simulink model "Simulateur_VRemise_eq06"  (R2024a)
settings: Solver=ode4  StartTime=0.0  StopTime=3  FixedStep=1e-06  RelTol=1e-3
InitFcn:
  | Init
values from neighbouring files (symbols this model uses):
  adL0 = -9.95e-3    (= -0.00995)    [Init.m]    (also in Init_Complet.m = -9.95e-06)
  adL1 = -9.10e-3    (= -0.0091)    [Init.m]    (also in Init_Complet.m = -9.1e-06)
  aKb0 = -1.41e-2    (= -0.0141)    [Init.m]    (also in Init_Complet.m)
  aKb1 = 5.96e-5    (= 5.96e-05)    [Init.m]    (also in Init_Complet.m)
  aL0 = 1.1256e-3    (= 0.0011256)    [Init.m]    (also in Init_Complet.m)
  aL1 = -9.95e-6    (= -9.95e-06)    [Init.m]    (also in Init_Complet.m)
  aL2 = -4.55e-6    (= -4.55e-06)    [Init.m]    (also in Init_Complet.m)
  aPhi0 = -1.41e-2    (= -0.0141)    [Init.m]    (also in Init_Complet.m)
  aPhi1 = 5.96e-5    (= 5.96e-05)    [Init.m]    (also in Init_Complet.m)
  b = 72.82e-3    (= 0.07282)    [Init.m]    (also in Init_Complet.m)
  Ccmax = 5    [Init.m]    (also in Init_Complet.m)
  Ccmin = 0    [Init.m]    (also in Init_Complet.m)
  Ccoff = 2.5    [Init.m]    (also in Init_Complet.m)
  d = 1850    [Init.m]    (also in Init_Complet.m)
  dt = 5e-6    (= 5e-06)    [Init.m]    (also in Init_Complet.m)
  E = 18.6e9    (= 18600000000)    [Init.m]    (also in Init_Complet.m)
  h = 1.46e-3    (= 0.00146)    [Init.m]    (also in Init_Complet.m)
  Imoff = 2.5    [Init.m]    (also in Init_Complet.m)
  K_pwm = 1/5    (= 0.2)    [Init.m]    (also in Init_Complet.m)
  KampL = 1    [Init.m]    (also in Init_Complet.m)
  Kd_pos = 0.00000405    (= 4.05e-06)    [Init.m]    (also in Init_Complet.m = 0.017)
  Ki_i = 180    [Init.m]    (also in Init_Complet.m)
  Ki_pos = 1.2    [Init.m]    (also in Init_Complet.m = 2.8333)
  Km = 1/1.1    (= 0.909090909091)    [Init.m]    (also in Init_Complet.m)
  Kp_i = 0.18    [Init.m]    (also in Init_Complet.m)
  Kp_pos = 0.005    [Init.m]    (also in Init_Complet.m = 0.85)
  Kpos = 205    [Init.m]    (also in Init_Complet.m)
  Kpwmo = 5    [Init.m]    (also in Init_Complet.m)
  Ksh = 1    [Init.m]    (also in Init_Complet.m)
  L = 25e-2    (= 0.25)    [Init.m]    (also in Init_Complet.m)
  M_l_p_b = 0.137    [Init.m]    (also in Init_Complet.m)
  N = 22    [Init.m]    (also in Init_Complet.m)
  Offp = 2.3025    [Init.m]    (also in Init_Complet.m)
  q = 0.14    [Init.m]    (also in Init_Complet.m)
  Rb = 1.63    [Init.m]    (also in Init_Complet.m)
  Ts_p = Ts_reg    (= 1e-06)    [Init.m]    (also in Init_Complet.m = 0.002)
  Vamp_max = 5    [Init.m]    (also in Init_Complet.m)
  Vamp_min = 0    [Init.m]    (also in Init_Complet.m)
  Vmoff = 2.5    [Init.m]    (also in Init_Complet.m)
  Vref = 1.8    [Init.m]    (also in Init_Complet.m)
  zeta = 0.0917    [Init.m]    (also in Init_Complet.m)
libraries: simulink x3, slpidlib x2
settings Model: SimulationMode=accelerator  Creator=jeann  LastModifiedBy=jotur116
settings RTWCC: GPUComputeCapability=3.5

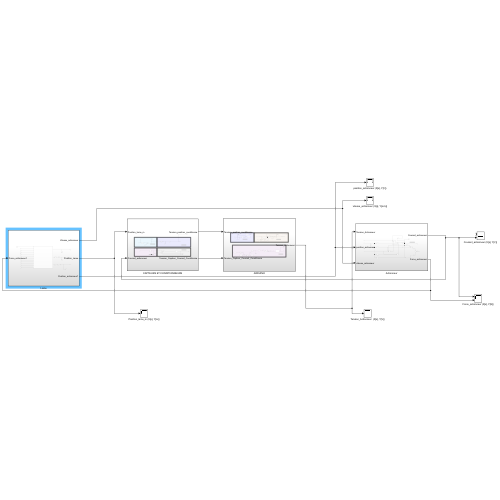
[thumbnail: Simulink's stored preview of the top-level diagram]
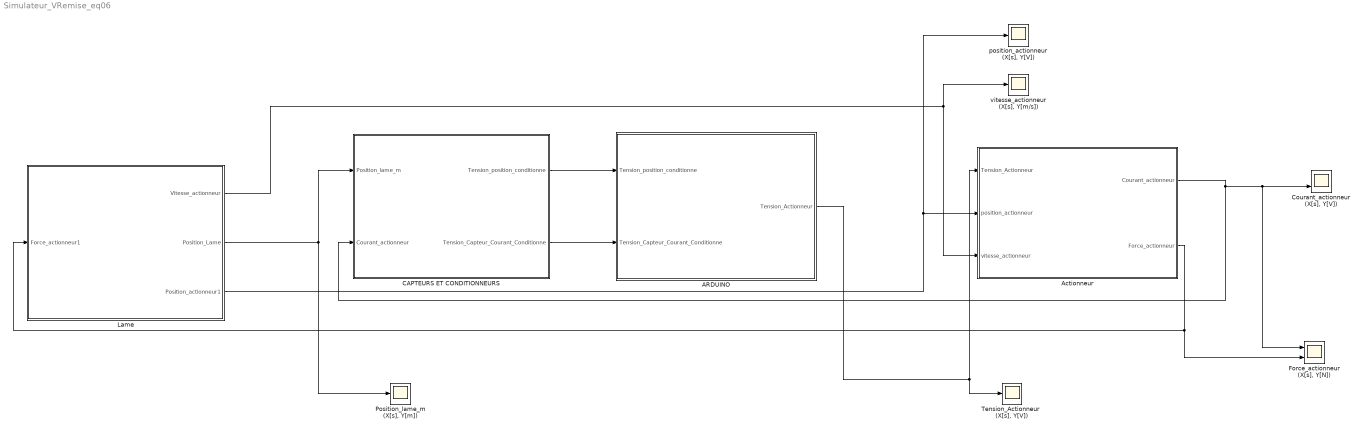
== system Simulateur_VRemise_eq06 ==
  ARDUINO : Subsystem
  Actionneur : Subsystem
  CAPTEURS ET CONDITIONNEURS : Subsystem
  "Courant_actionneur (X[s], Y[V])" : Scope  NumInputPorts=2
  "Force_actionneur (X[s], Y[N])" : Scope  NumInputPorts=2
  Lame : Subsystem
  "Position_lame_m (X[s], Y[m])" : Scope
  "Tension_Actionneur  (X[s], Y[V])" : Scope
  "position_actionneur (X[s], Y[V])" : Scope
  "vitesse_actionneur (X[s], Y[m/s])" : Scope
  wires:
  Lame/3(Position_actionneur1) -> "position_actionneur (X[s], Y[V])"/1, Actionneur/2(position_actionneur)
  Lame/1(Vitesse_actionneur) -> Actionneur/3(vitesse_actionneur), "vitesse_actionneur (X[s], Y[m/s])"/1
  Lame/2(Position_Lame) -> CAPTEURS ET CONDITIONNEURS/1(Position_lame_m), "Position_lame_m (X[s], Y[m])"/1
  CAPTEURS ET CONDITIONNEURS/1(Tension_position_conditionne) -> ARDUINO/1(Tension_position_conditionne)
  CAPTEURS ET CONDITIONNEURS/2(Tension_Capteur_Courant_Conditionne) -> ARDUINO/2(Tension_Capteur_Courant_Conditionne)
  ARDUINO/1(Tension_Actionneur) -> "Tension_Actionneur  (X[s], Y[V])"/1, Actionneur/1(Tension_Actionneur)
  Actionneur/1(Courant_actionneur) -> CAPTEURS ET CONDITIONNEURS/2(Courant_actionneur), "Courant_actionneur (X[s], Y[V])"/2, "Force_actionneur (X[s], Y[N])"/1
  Actionneur/2(Force_actionneur) -> Lame/1(Force_actionneur1), "Force_actionneur (X[s], Y[N])"/2

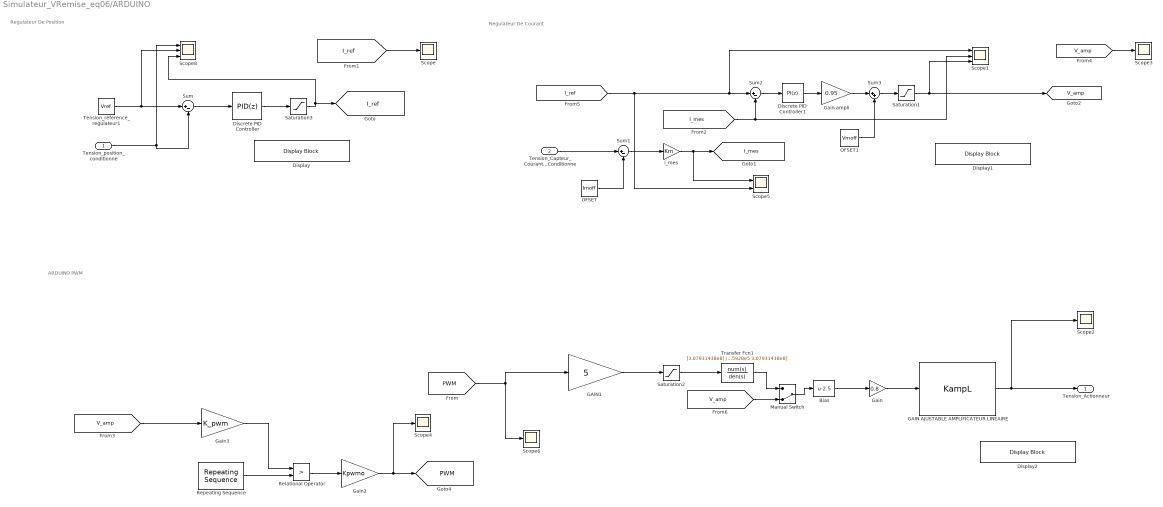
== system Simulateur_VRemise_eq06/ARDUINO ==
  note: Regulateur De Position
  note: Regulateur De Courant
  note: ARDUINO PWM
  Tension_position_conditionne : Inport
  Tension_Capteur_Courant_Conditionne : Inport  Port=2
  Bias : Bias  Bias=-2.5  SaturateOnIntegerOverflow=off
  Discrete PID Controller : slpidlib/PID Controller  Controller=PID  Form=Parallel  TimeDomain=Discrete-time  UseExternalTs=off  SampleTime=Ts_p  IntegratorMethod=Forward Euler  FilterMethod=Forward Euler  ControllerParametersSource=internal  P=Kp_pos  I=Ki_pos  UseKiTs=off  D=Kd_pos  UseExternalDerivativeSource=off  N=100  UseFilter=on  TunerSelectOption=Transfer Function Based (PID Tuner App)  InitialConditionSource=internal  InitialConditionForIntegrator=0  InitialConditionForFilter=0  DifferentiatorICPrevScaledInput=0  ExternalReset=none  TrackingMode=off  Kt=1  LimitOutput=on  SatLimitsSource=internal  UpperSaturationLimit=2.35  LowerSaturationLimit=-2.35  LinearizeAsGain=off  AntiWindupMode=back-calculation  Kb=1  LimitIntegrator=off  UpperIntegratorSaturationLimit=inf  LowerIntegratorSaturationLimit=-inf  POutMin=[]  POutMax=[]  IOutMin=[]  IOutMax=[]  DOutMin=[]  DOutMax=[]  NOutMin=[]  NOutMax=[]  SumOutMin=[]  SumOutMax=[]  SaturationOutMin=[]  SaturationOutMax=[]  PParamMin=[]  PParamMax=[]  IParamMin=[]  IParamMax=[]  DParamMin=[]  DParamMax=[]  NParamMin=[]  NParamMax=[]  KbParamMin=[]  KbParamMax=[]  KtParamMin=[]  KtParamMax=[]  KbOutMin=[]  KbOutMax=[]  KtOutMin=[]  KtOutMax=[]  IntegratorOutMin=[]  IntegratorOutMax=[]  FilterOutMin=[]  FilterOutMax=[]  SumI1OutMin=[]  SumI1OutMax=[]  SumI2OutMin=[]  SumI2OutMax=[]  SumI3OutMin=[]  SumI3OutMax=[]  SumI4OutMin=[]  SumI4OutMax=[]  SumDOutMin=[]  SumDOutMax=[]  DifferentiatorOutMin=[]  DifferentiatorOutMax=[]  FilterDiffOutCoefMin=[]  FilterDiffOutCoefMax=[]  ReciprocalOutMin=[]  ReciprocalOutMax=[]  SumDenOutMin=[]  SumDenOutMax=[]  SumNumOutMin=[]  SumNumOutMax=[]  DivideOutMin=[]  DivideOutMax=[]  UdiffTsProdOutMin=[]  UdiffTsProdOutMax=[]  NTsProdOutMin=[]  NTsProdOutMax=[]  UintegralTsProdOutMin=[]  UintegralTsProdOutMax=[]  UngainTsProdOutMin=[]  UngainTsProdOutMax=[]  ClampingZeroOutDataTypeStr=Inherit: Inherit via back propagation  ClampingZeroOutMin=[]  ClampingZeroOutMax=[]  FilterDenConstantOutDataTypeStr=Inherit: Inherit via back propagation  FilterDenConstantOutMin=[]  FilterDenConstantOutMax=[]  PCopyOutDataTypeStr=Inherit: Inherit via back propagation  PCopyOutMin=[]  PCopyOutMax=[]  NCopyOutDataTypeStr=Inherit: Inherit via back propagation  NCopyOutMin=[]  NCopyOutMax=[]  IntegratorContinuousStateAttributes=''  IntegratorStateMustResolveToSignalObject=off  IntegratorRTWStateStorageClass=Auto  FilterContinuousStateAttributes=''  FilterStateMustResolveToSignalObject=off  FilterRTWStateStorageClass=Auto  ParallelPVariant=InternalParameters  IdealPVariant=Disabled  IVariant=InternalParameters  DVariant=InternalParameters  IntegratorVariant=Discrete  SatVariant=Enabled  AWVariant=BackCalculation  PCopyVariant=Disabled  TRVariant=Disabled  FdbkBlocksVariant=Forward  IdealPFdbkVariant=Disabled  SatFdbkVariant=Disabled  DerivativeFilterVariant=ForwardEulerFilter  NVariant=InternalParameters  NCopyVariant=Disabled  FilterICVariant=InternalICsFilter  IntegratorICVariant=InternalICs  ExternalResetVariant=Disabled  TRSumVariant=Passthrough  SumFdbkVariant=Disabled  SumVariant=Sum_PID  TsampFilterVariant=InternalTs  TsampNgainVariant=Passthrough  TsampIntegralVariant=Disabled_SignalSpec  ExternalSaturationOutDataTypeStr=Inherit: Same as second input  DerivativeSourceVariant=ErrorSignal
      settings: LibrarySourceBlock=simulink/Discrete/Discrete PID Controller
  Discrete PID Controller1 : slpidlib/PID Controller  Controller=PI  Form=Parallel  TimeDomain=Discrete-time  UseExternalTs=off  SampleTime=0.002  IntegratorMethod=Forward Euler  FilterMethod=Forward Euler  ControllerParametersSource=internal  P=Kp_i  I=Ki_i  UseKiTs=off  D=0  UseExternalDerivativeSource=off  N=100  UseFilter=on  TunerSelectOption=Transfer Function Based (PID Tuner App)  InitialConditionSource=internal  InitialConditionForIntegrator=0  InitialConditionForFilter=0  DifferentiatorICPrevScaledInput=0  ExternalReset=none  TrackingMode=off  Kt=1  LimitOutput=off  SatLimitsSource=internal  UpperSaturationLimit=5  LowerSaturationLimit=0  LinearizeAsGain=off  AntiWindupMode=back-calculation  Kb=1  LimitIntegrator=off  UpperIntegratorSaturationLimit=inf  LowerIntegratorSaturationLimit=-inf  POutMin=[]  POutMax=[]  IOutMin=[]  IOutMax=[]  DOutMin=[]  DOutMax=[]  NOutMin=[]  NOutMax=[]  SumOutMin=[]  SumOutMax=[]  SaturationOutMin=[]  SaturationOutMax=[]  PParamMin=[]  PParamMax=[]  IParamMin=[]  IParamMax=[]  DParamMin=[]  DParamMax=[]  NParamMin=[]  NParamMax=[]  KbParamMin=[]  KbParamMax=[]  KtParamMin=[]  KtParamMax=[]  KbOutMin=[]  KbOutMax=[]  KtOutMin=[]  KtOutMax=[]  IntegratorOutMin=[]  IntegratorOutMax=[]  FilterOutMin=[]  FilterOutMax=[]  SumI1OutMin=[]  SumI1OutMax=[]  SumI2OutMin=[]  SumI2OutMax=[]  SumI3OutMin=[]  SumI3OutMax=[]  SumI4OutMin=[]  SumI4OutMax=[]  SumDOutMin=[]  SumDOutMax=[]  DifferentiatorOutMin=[]  DifferentiatorOutMax=[]  FilterDiffOutCoefMin=[]  FilterDiffOutCoefMax=[]  ReciprocalOutMin=[]  ReciprocalOutMax=[]  SumDenOutMin=[]  SumDenOutMax=[]  SumNumOutMin=[]  SumNumOutMax=[]  DivideOutMin=[]  DivideOutMax=[]  UdiffTsProdOutMin=[]  UdiffTsProdOutMax=[]  NTsProdOutMin=[]  NTsProdOutMax=[]  UintegralTsProdOutMin=[]  UintegralTsProdOutMax=[]  UngainTsProdOutMin=[]  UngainTsProdOutMax=[]  ClampingZeroOutDataTypeStr=Inherit: Inherit via back propagation  ClampingZeroOutMin=[]  ClampingZeroOutMax=[]  FilterDenConstantOutDataTypeStr=Inherit: Inherit via back propagation  FilterDenConstantOutMin=[]  FilterDenConstantOutMax=[]  PCopyOutDataTypeStr=Inherit: Inherit via back propagation  PCopyOutMin=[]  PCopyOutMax=[]  NCopyOutDataTypeStr=Inherit: Inherit via back propagation  NCopyOutMin=[]  NCopyOutMax=[]  IntegratorContinuousStateAttributes=''  IntegratorStateMustResolveToSignalObject=off  IntegratorRTWStateStorageClass=Auto  FilterContinuousStateAttributes=''  FilterStateMustResolveToSignalObject=off  FilterRTWStateStorageClass=Auto  ParallelPVariant=InternalParameters  IdealPVariant=Disabled  IVariant=InternalParameters  DVariant=Disabled  IntegratorVariant=Discrete  SatVariant=Disabled  AWVariant=Passthrough  PCopyVariant=Disabled  TRVariant=Disabled  FdbkBlocksVariant=Forward  IdealPFdbkVariant=Disabled  SatFdbkVariant=Disabled  DerivativeFilterVariant=Disabled  NVariant=Disabled  NCopyVariant=Disabled_SignalSpec  FilterICVariant=Disabled  IntegratorICVariant=InternalICs  ExternalResetVariant=Disabled  TRSumVariant=Passthrough  SumFdbkVariant=Disabled  SumVariant=Sum_PI  TsampFilterVariant=InternalTs  TsampNgainVariant=Passthrough  TsampIntegralVariant=Disabled_SignalSpec  ExternalSaturationOutDataTypeStr=Inherit: Same as second input  DerivativeSourceVariant=Disabled
      settings: LibrarySourceBlock=simulink/Discrete/Discrete PID Controller
  Display : DisplayBlock  LabelPosition=Hide  Transparency=1
  Display1 : DisplayBlock  LabelPosition=Hide  Transparency=1
  Display2 : DisplayBlock  LabelPosition=Hide  Transparency=1
  GAIN AJUSTABLE AMPLIFICATEUR LINEAIRE : simulink/Math Operations/Slider Gain  gain=KampL  low=1  high=5
  GAIN1 : Gain  Gain=5
  Gain : Gain  Gain=0.8
  "Gain ampli " : Gain  Gain=0.95
  Gain2 : Gain  Gain=Kpwmo  ParamDataTypeStr=double
  Gain3 : Gain  Gain=K_pwm
  Manual Switch : ManualSwitch  CurrentSetting=0
  OFSET : Constant  Value=Imoff
  OFSET1 : Constant  Value=Vmoff
  Relational Operator : RelationalOperator  Operator=>  OutDataTypeStr=boolean  RndMeth=Simplest  InputSameDT=off
  Repeating Sequence : simulink/Sources/Repeating Sequence  rep_seq_t=[0 3.2e-5 6.4e-5]  rep_seq_y=[0 1 0]
  Saturation1 : Saturate  UpperLimit=Vamp_max  LowerLimit=Vamp_min
  Saturation2 : Saturate  UpperLimit=Vamp_max  LowerLimit=Vamp_min
  Saturation3 : Saturate  UpperLimit=2.35  LowerLimit=-2.35
  Scope{,2..4,6} (5 alike) : Scope
  Scope1 : Scope  NumInputPorts=3
  Scope5 : Scope  NumInputPorts=2
  Scope8 : Scope  NumInputPorts=3
  Sum : Sum  Inputs=|+-
  Sum1 : Sum  Inputs=|+-
  Sum2 : Sum  Inputs=|+-
  Sum3 : Sum  Inputs=|++
  Tension_reference_regulateur1 : Constant  Value=Vref
  Transfer Fcn1 : TransferFcn  Numerator=[3.07931438e8]  Denominator=[1 1.0115928e5 3.07931438e8]
  i_mes : Gain  Gain=Km
  Tension_Actionneur : Outport
  tag scope: I_mes=global, I_ref=global, PWM=global, V_amp=global
  wires:
  [I_ref] -> Scope/1
  Discrete PID Controller/1 -> Saturation3/1
  Sum1/1 -> i_mes/1
  Discrete PID Controller1/1 -> "Gain ampli "/1
  "Gain ampli "/1 -> Sum3/1
  Sum2/1 -> Discrete PID Controller1/1
  i_mes/1 -> Scope5/1, [I_mes]
  [V_amp] -> Scope3/1
  OFSET/1 -> Sum1/2
  OFSET1/1 -> Sum3/2
  Sum3/1 -> Saturation1/1
  Tension_Capteur_Courant_Conditionne/1 -> Sum1/1
  Gain2/1 -> Scope4/1, [PWM]
  Gain3/1 -> Relational Operator/1
  Repeating Sequence/1 -> Relational Operator/2
  Relational Operator/1 -> Gain2/1
  [V_amp] -> Gain3/1
  [PWM] -> Scope6/1, GAIN1/1
  [I_ref] -> Scope5/2, Scope1/1, Sum2/1
  [I_mes] -> Scope1/2, Sum2/2
  Saturation1/1 -> [V_amp], Scope1/3
  Saturation3/1 -> [I_ref], Scope8/3
  GAIN AJUSTABLE AMPLIFICATEUR LINEAIRE/1 -> Tension_Actionneur/1, Scope2/1
  Sum/1 -> Discrete PID Controller/1
  Tension_position_conditionne/1 -> Scope8/1, Sum/2
  Tension_reference_regulateur1/1 -> Scope8/2, Sum/1
  GAIN1/1 -> Saturation2/1
  Saturation2/1 -> Transfer Fcn1/1
  Bias/1 -> Gain/1
  Gain/1 -> GAIN AJUSTABLE AMPLIFICATEUR LINEAIRE/1
  Transfer Fcn1/1 -> Manual Switch/1
  Manual Switch/1 -> Bias/1
  [V_amp] -> Manual Switch/2

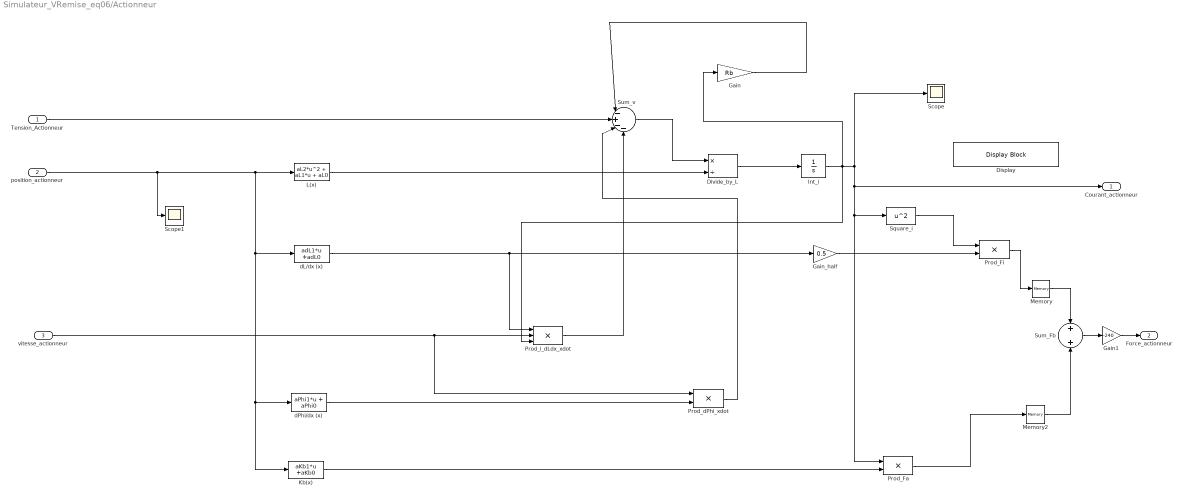
== system Simulateur_VRemise_eq06/Actionneur ==
  Tension_Actionneur : Inport
  position_actionneur : Inport  Port=2
  vitesse_actionneur : Inport  Port=3
  Display : DisplayBlock  LabelPosition=Hide  Transparency=1
  Divide_by_L : Product  Inputs=*/
  Gain : Gain  Gain=Rb
  Gain1 : Gain  Gain=-240
  Gain_half : Gain  Gain=0.5
  Int_i : Integrator
  Kb(x) : Fcn  Expr=aKb1*u +aKb0
  L(x) : Fcn  Expr=aL2*u^2 + aL1*u + aL0
  Memory : Memory
  Memory2 : Memory
  Prod_Fa : Product
  Prod_Fi : Product
  Prod_dPhi_xdot : Product
  Prod_i_dLdx_xdot : Product  Inputs=3
  Scope : Scope
  Scope1 : Scope
  Square_i : Math  Operator=square
  Sum_Fb : Sum
  Sum_v : Sum  Inputs=|-+--
  dL/dx (x) : Fcn  Expr=adL1*u +adL0
  dPhi/dx (x) : Fcn  Expr=aPhi1*u + aPhi0
  Courant_actionneur : Outport
  Force_actionneur : Outport  Port=2
  wires:
  dL/dx (x)/1 -> Gain_half/1, Prod_i_dLdx_xdot/1
  Sum_Fb/1 -> Gain1/1
  Gain/1 -> Sum_v/1
  Prod_i_dLdx_xdot/1 -> Sum_v/4
  L(x)/1 -> Divide_by_L/2
  Square_i/1 -> Prod_Fi/1
  Prod_dPhi_xdot/1 -> Sum_v/3
  Gain_half/1 -> Prod_Fi/2
  dPhi/dx (x)/1 -> Prod_dPhi_xdot/2
  Divide_by_L/1 -> Int_i/1
  Int_i/1 -> Prod_i_dLdx_xdot/3, Courant_actionneur/1, Square_i/1, Prod_Fa/1, Scope/1, Gain/1
  Sum_v/1 -> Divide_by_L/1
  vitesse_actionneur/1 -> Prod_dPhi_xdot/1, Prod_i_dLdx_xdot/2
  Kb(x)/1 -> Prod_Fa/2
  position_actionneur/1 -> Scope1/1, dL/dx (x)/1, Kb(x)/1, dPhi/dx (x)/1, L(x)/1
  Tension_Actionneur/1 -> Sum_v/2
  Prod_Fi/1 -> Memory/1
  Memory/1 -> Sum_Fb/1
  Prod_Fa/1 -> Memory2/1
  Memory2/1 -> Sum_Fb/2
  Gain1/1 -> Force_actionneur/1

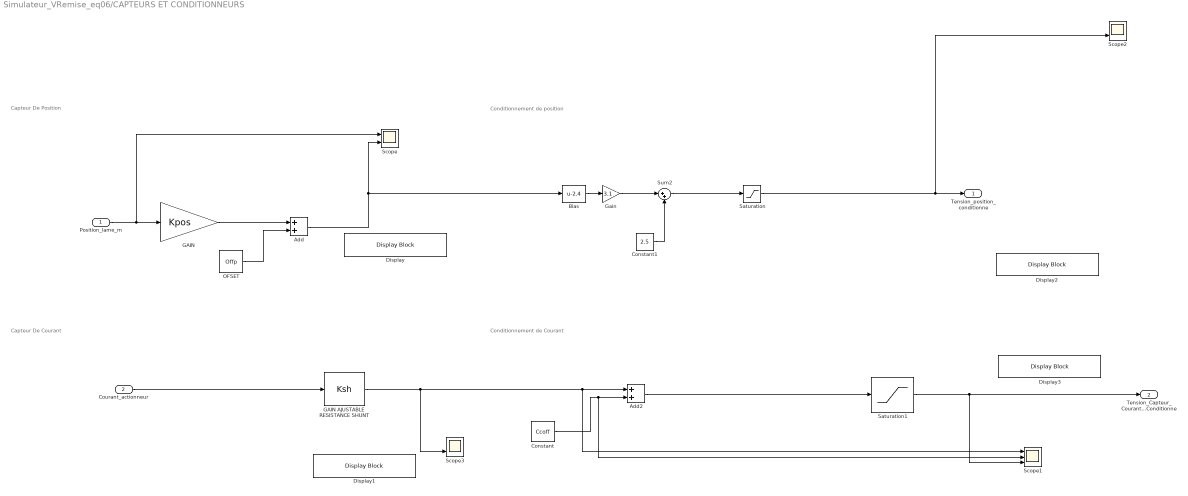
== system Simulateur_VRemise_eq06/CAPTEURS ET CONDITIONNEURS ==
  note: Capteur De Position
  note: Conditionnement de position
  note: Capteur De Courant
  note: Conditionnement de Courant
  Position_lame_m : Inport
  Courant_actionneur : Inport  Port=2
  Add : Sum
  Add2 : Sum
  Bias : Bias  Bias=-2.4  SaturateOnIntegerOverflow=off
  Constant : Constant  Value=Ccoff
  Constant1 : Constant  Value=2.5
  Display{,1..3} (4 alike) : DisplayBlock  LabelPosition=Hide  Transparency=1
  GAIN : Gain  Gain=Kpos
  GAIN AJUSTABLE RESISTANCE SHUNT : simulink/Math Operations/Slider Gain  gain=Ksh  low=1  high=10
  Gain : Gain  Gain=3.1
  OFSET : Constant  Value=Offp
  Saturation : Saturate  UpperLimit=5  LowerLimit=0
  Saturation1 : Saturate  UpperLimit=Ccmax  LowerLimit=Ccmin
  Scope : Scope  NumInputPorts=2
  Scope1 : Scope  NumInputPorts=3
  Scope2 : Scope  NumInputPorts=2
  Scope3 : Scope  NumInputPorts=2
  Sum2 : Sum  Inputs=|++
  Tension_position_conditionne : Outport
  Tension_Capteur_Courant_Conditionne : Outport  Port=2
  wires:
  GAIN/1 -> Add/1
  OFSET/1 -> Add/2
  Saturation1/1 -> Tension_Capteur_Courant_Conditionne/1, Scope1/3
  Position_lame_m/1 -> Scope/1, GAIN/1
  GAIN AJUSTABLE RESISTANCE SHUNT/1 -> Scope1/1, Add2/1, Scope3/2
  Constant/1 -> Scope1/2, Add2/2
  Gain/1 -> Sum2/1
  Constant1/1 -> Sum2/2
  Sum2/1 -> Saturation/1
  Saturation/1 -> Tension_position_conditionne/1, Scope2/2
  Add2/1 -> Saturation1/1
  Courant_actionneur/1 -> GAIN AJUSTABLE RESISTANCE SHUNT/1
  Add/1 -> Bias/1, Scope/2
  Bias/1 -> Gain/1

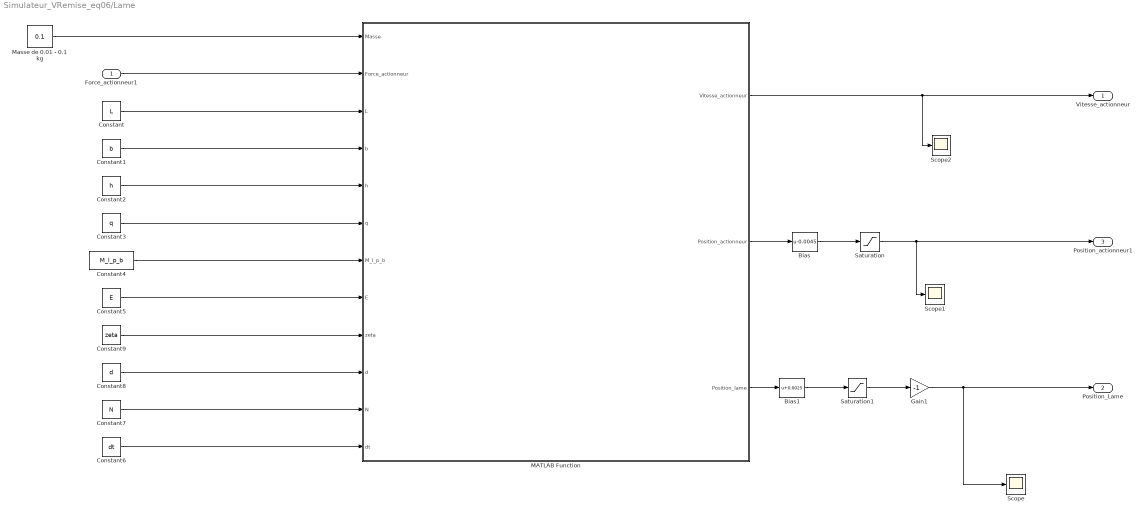
== system Simulateur_VRemise_eq06/Lame ==
  Force_actionneur1 : Inport
  Bias : Bias  Bias=-0.0045  SaturateOnIntegerOverflow=off
  Bias1 : Bias  Bias=0.0025  SaturateOnIntegerOverflow=off
  Constant : Constant  Value=L
  Constant1 : Constant  Value=b
  Constant2 : Constant  Value=h
  Constant3 : Constant  Value=q
  Constant4 : Constant  Value=M_l_p_b
  Constant5 : Constant  Value=E
  Constant6 : Constant  Value=dt
  Constant7 : Constant  Value=N
  Constant8 : Constant  Value=d
  Constant9 : Constant  Value=zeta
  Gain1 : Gain  Gain=-1
  MATLAB Function : MATLAB Function  TreatAsAtomicUnit=on
  Masse de 0.01 - 0.1 kg : Constant  Value=0.1
  Saturation : Saturate  UpperLimit=0.003  LowerLimit=-0.002
  Saturation1 : Saturate  UpperLimit=0.003  LowerLimit=-0.004
  Scope : Scope
  Scope1 : Scope
  Scope2 : Scope
  Vitesse_actionneur : Outport
  Position_Lame : Outport  Port=2
  Position_actionneur1 : Outport  Port=3
  wires:
  Constant7/1 -> MATLAB Function/11(N)
  Constant3/1 -> MATLAB Function/6(q)
  Constant8/1 -> MATLAB Function/10(d)
  Constant1/1 -> MATLAB Function/4(b)
  Constant2/1 -> MATLAB Function/5(h)
  Constant5/1 -> MATLAB Function/8(E)
  Force_actionneur1/1 -> MATLAB Function/2(Force_actionneur)
  Constant4/1 -> MATLAB Function/7(M_l_p_b)
  MATLAB Function/1(Vitesse_actionneur) -> Scope2/1, Vitesse_actionneur/1
  MATLAB Function/2(Position_actionneur) -> Bias/1
  Masse de 0.01 - 0.1 kg/1 -> MATLAB Function/1(Masse)
  Constant9/1 -> MATLAB Function/9(zeta)
  Constant/1 -> MATLAB Function/3(L)
  Constant6/1 -> MATLAB Function/12(dt)
  MATLAB Function/3(Position_lame) -> Bias1/1
  Bias1/1 -> Saturation1/1
  Bias/1 -> Saturation/1
  Saturation/1 -> Scope1/1, Position_actionneur1/1
  Saturation1/1 -> Gain1/1
  Gain1/1 -> Position_Lame/1, Scope/1

== matlab function Simulateur_VRemise_eq06/Lame/MATLAB Function ==
  data: Masse input; Vitesse_actionneur output; Force_actionneur input; L input; b input; h input; q input; M_l_p_b input; E input; zeta input; d input; N input; dt input; Position_actionneur output; Position_lame output
function [Vitesse_actionneur, Position_actionneur, Position_lame] = ...
    ModeleLame(Masse, Force_actionneur, L, b, h, q, M_l_p_b, E, zeta, d, N, dt)
%#codegen
%
%%----------------------------------------------------------
% Parametres :
%----------------------------------------------------------
%   L                 [m]   : longueur de la lame
%   b                 [m]   : largeur de la lame
%   h                 [m]   : epaisseur de la lame
%   q                 [m]   : position du centre du plateau
%   M_l_p_b           [kg]  : masse totale lame + plateau + bobine
%   E                 [Pa]  : module de Young
%   zeta              [-]   : amortissement equivalent
%   d                 [kg/m^3] : densite
%   N                 [-]   : nombre de noeuds physiques
%   dt                [s]   : pas de temps
%
%
%----------------------------------------------------------
% Entrees :
%----------------------------------------------------------
%   Masse             [kg]  : masse ajoutee sur le plateau
%   Force_actionneur  [N]   : force appliquee par l'actionneur
%
%
%----------------------------------------------------------
% Sorties :
%----------------------------------------------------------
%   Vitesse_actionneur   [m/s] : vitesse au centre du plateau
%   Position_actionneur  [m] : position au centre du plateau
%   Position_lame        [m] : position a l'extremite libre

MAXN = 64;

persistent w w_old initialized N_old first_output_done

if isempty(initialized)
    w = zeros(1, MAXN);
    w_old = zeros(1, MAXN);
    initialized = true;
    N_old = int32(-1);
    first_output_done = false;
end

%% Parametres prototype
g = 9.81;

% Plateau + bobine
l_plateau = 0.06;      % [m]
m_plateau = 0.038;     % [kg]
m_bobine  = 0.031;     % [kg]

% Offset statique de la lame pour recentrer la sortie autour de zero
offset_lame = 11.9e-3;  % [m]

%% Securite sur N
N = int32(N);

if N < int32(8)
    N = int32(8);
end

if N > int32(MAXN - 2)
    N = int32(MAXN - 2);
end

if N_old ~= N
    w(:) = 0.0;
    w_old(:) = 0.0;
    N_old = N;
    first_output_done = false;
end

%% Geometrie et matiere
J  = b * h^3 / 12.0;      % moment quadratique
mu = d * b * h;           % masse lineique lame nue [kg/m]

nx_phys = double(N);
dx = L / (nx_phys - 1.0);

% 2 noeuds fantomes
nx = N + int32(2);

%% Position du plateau (centre)
q_centre = q;

if q_centre < 0.0
    q_centre = 0.0;
elseif q_centre > L
    q_centre = L;
end

idx_centre = int32(round(q_centre / dx)) + int32(2);

if idx_centre < int32(3)
    idx_centre = int32(3);
elseif idx_centre > nx - int32(2)
    idx_centre = nx - int32(2);
end

%% Zone occupee par le plateau
nb_dx_plateau = int32(round(l_plateau / dx));
if nb_dx_plateau < int32(1)
    nb_dx_plateau = int32(1);
end

demi_largeur = idivide(nb_dx_plateau, int32(2), 'floor');

i_debut = idx_centre - demi_largeur;
i_fin   = idx_centre + demi_largeur;

if i_debut < int32(3)
    i_debut = int32(3);
end

if i_fin > nx - int32(2)
    i_fin = nx - int32(2);
end

l_plateau_simul = double(i_fin - i_debut + int32(1)) * dx;

%% Masse lame / plateau / bobine
M_lame_calc = mu * L;

% Verif douce avec la masse totale fournie
M_plateau_bobine_geom = m_plateau + m_bobine;
M_plateau_bobine_tot  = M_l_p_b - M_lame_calc;

if M_plateau_bobine_tot > 0.0
    M_plateau_bobine = M_plateau_bobine_tot;
else
    M_plateau_bobine = M_plateau_bobine_geom;
end

M_charge = Masse;
if M_charge < 0.0
    M_charge = 0.0;
end

%% Vecteur de masse lineique
mu_vect = mu * ones(1, MAXN);

% Masse supplementaire repartie sur la zone du plateau
mu_sup = (M_plateau_bobine + M_charge) / l_plateau_simul;

for k = i_debut:i_fin
    mu_vect(k) = mu + mu_sup;
end

%% Amortissement equivalent distribue
omega_1 = sqrt(((1.8751 / L)^4) * (E * J / mu));
beta    = 2.0 * mu * zeta * omega_1;

%% Coefficients locaux
coeff1 = zeros(1, MAXN);
coeff2 = zeros(1, MAXN);
coeff3 = zeros(1, MAXN);
coeff4 = zeros(1, MAXN);

dx_n = dx / L;

for k = int32(1):nx
    mu_simu_k = sqrt((E * J) / (mu_vect(k) * L^4)) * (dt / (dx_n^2));

    coeff1(k) = 2.0 - ((beta * dt) / mu_vect(k)) - 6.0 * mu_simu_k^2;
    coeff2(k) = 4.0 * mu_simu_k^2;
    coeff3(k) = -mu_simu_k^2;
    coeff4(k) = ((beta * dt) / mu_vect(k)) - 1.0;
end

%% Forces reparties
F_vect = zeros(1, MAXN);

% Poids propre sur toute la lame
for k = int32(1):nx
    F_vect(k) = -g * mu_vect(k);
end

% Force actionneur + poids de la charge sur la zone du plateau
F_zone = (Force_actionneur) / l_plateau_simul;

for k = i_debut:i_fin
    F_vect(k) = F_vect(k) + F_zone;
end

%% Terme de force
coeff_force = zeros(1, MAXN);
for k = int32(1):nx
    coeff_force(k) = (dt^2 / mu_vect(k)) * F_vect(k);
end

%% Mise a jour dynamique
w_new = zeros(1, MAXN);

for i = int32(3):nx - int32(2)
    w_new(i) = coeff1(i) * w(i) ...
             + coeff2(i) * (w(i+1) + w(i-1)) ...
             + coeff3(i) * (w(i+2) + w(i-2)) ...
             + coeff4(i) * w_old(i) ...
             + coeff_force(i);
end

%% Conditions aux limites
% Encastrement a gauche
w_new(1) = 0.0;
w_new(2) = 0.0;

% Extremite libre a droite
w_new(nx - int32(1)) = 2.0 * w_new(nx - int32(2)) - w_new(nx - int32(3));
w_new(nx)            = 2.0 * w_new(nx - int32(1)) - w_new(nx - int32(2));

%% Sorties
Position_actionneur = -w_new(idx_centre);
Vitesse_actionneur  = -(w_new(idx_centre) - w(idx_centre)) / dt;
Position_lame       = -w_new(nx - int32(1)) - offset_lame;

% Forcer uniquement le tout premier echantillon de Position_lame a zero
if ~first_output_done
    Position_lame = 0.0;
    first_output_done = true;
end

%% Mise a jour memoire
w_old = w;
w = w_new;

end
